simulink model "untitled"  (R2019b)
settings: Solver=VariableStepAuto  StartTime=0.0  StopTime=10.0  RelTol=1e-3
values from neighbouring files (symbols this model uses):
  Adz = (Ad+Bd*K)    [Untitled.m]
  Bdz = zeros(size(Bd))    [Untitled.m]
  K = -inv(R+Bd'*P*Bd)*Bd'*P*Ad    [Untitled.m]
  Ts = 0.2    [Untitled.m]
  x0k = [2 3 5]'    [Untitled.m]
undefined symbols (not defined in the file or in its folder): Ad, Bd
settings Model: Creator=patti  LastModifiedBy=patti

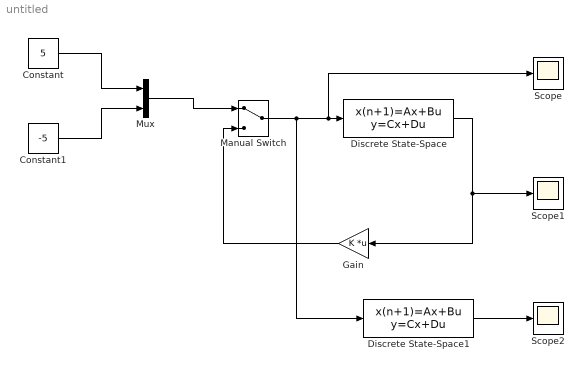
== system untitled ==
  Constant : Constant  Value=5
  Constant1 : Constant  Value=-5
  Discrete State-Space : DiscreteStateSpace  A=Ad  B=Bd  C=eye(3)  D=zeros(3,2)  InitialCondition=x0k  SampleTime=Ts
  Discrete State-Space1 : DiscreteStateSpace  A=Adz  B=Bdz  C=eye(3)  D=zeros(3,2)  InitialCondition=x0k  SampleTime=Ts
  Gain : Gain  Gain=K  Multiplication=Matrix(K*u)
  Manual Switch : ManualSwitch
  Mux : Mux  Inputs=2
  Scope : Scope
  Scope1 : Scope
  Scope2 : Scope
  wires:
  Constant/1 -> Mux/1
  Constant1/1 -> Mux/2
  Mux/1 -> Manual Switch/1
  Gain/1 -> Manual Switch/2
  Manual Switch/1 -> Scope/1, Discrete State-Space/1, Discrete State-Space1/1
  Discrete State-Space/1 -> Scope1/1, Gain/1
  Discrete State-Space1/1 -> Scope2/1
